simulink model "KalmanFilter_Corrected"  (R2024a)
settings: Solver=VariableStepDiscrete  StartTime=0.0  StopTime=100.0  RelTol=1e-3
values from neighbouring files (symbols this model uses):
  A = [1.1269, -0.4940, 0.1129 ... (first row only)    [KalmanFilter_Corrected_soc.m]
  B = [-0.3832,0,0 ... (first row only)    [KalmanFilter_Corrected_soc.m]
  C = [1;0;0]    [KalmanFilter_Corrected_soc.m]
  D = [0;0;0]    [KalmanFilter_Corrected_soc.m]
  P0 = eye(3)    [KalmanFilter_Corrected_soc.m]
  Q = 0    [KalmanFilter_Corrected_soc.m]
  R = [1,0, 0.1;0,0,0;0,0,0]    [KalmanFilter_Corrected_soc.m]
  X0 = [1; 0; 0]    [KalmanFilter_Corrected_soc.m]
undefined symbols (not defined in the file or in its folder): Discrete, Time
libraries: matrix_library x3, ctrlSharedLib x1
settings Model: Creator=Z634594  LastModifiedBy=DELL
settings SolverCC: AlgebraicLoopSolver=TrustRegion
settings DebuggingCC: UnconnectedInputMsg=warning  UnconnectedOutputMsg=warning  UnconnectedLineMsg=warning
settings ModelReferenceCC: EnableRefExpFcnMdlSchedulingChecks=on
settings SFSimCC: CustomCodeUndefinedFunction=UseInterfaceOnly
settings RTWCC: GPUComputeCapability=3.5

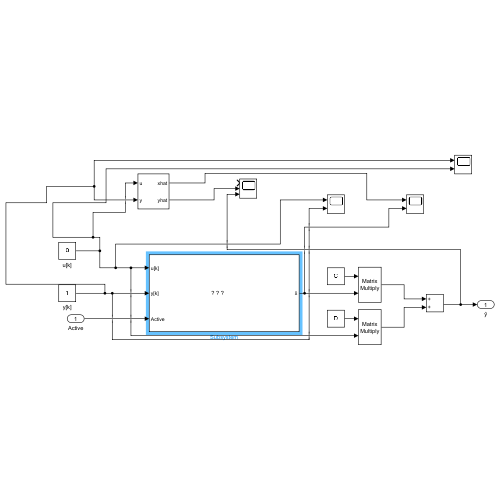
[thumbnail: Simulink's stored preview of the top-level diagram]
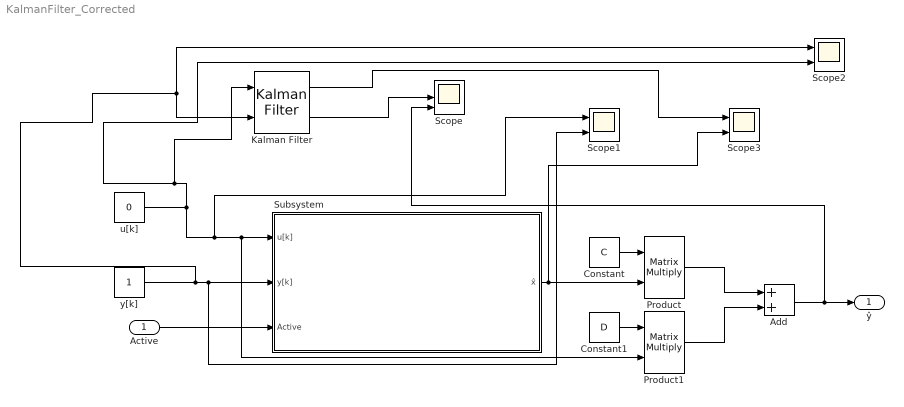
== system KalmanFilter_Corrected ==
  Active : Inport
  Add : Sum
  Constant : Constant  Value=C  VectorParams1D=off
  Constant1 : Constant  Value=D  VectorParams1D=off
  Kalman Filter : ctrlSharedLib/Kalman Filter  TimeDomain=Discrete-Time  UseCurrentEstimator=off  ModelSource=Individual A, B, C, D matrices  ModelSourceVariable=ss(0.95,1,1,0,1)  A=A  B=B  C=C  D=D  NumberOfStates=1  NumberOfInputs=1  NumberOfOutputs=1  InitialEstimateSource=Dialog  X0=[1; 0; 0];  P0=10  UseK=off  UseGH=off  NumberOfProcessNoiseInputs=1  G=1  TimeInvariantG=on  H=0  TimeInvariantH=on  Q=Q  TimeInvariantQ=on  R=1  TimeInvariantR=on  N=0  TimeInvariantN=on  AddInputPort=on  AddEnablePort=off  OutputEstimatedY=on  OutputP=off  Ts=-1
  Product : Product  Multiplication=Matrix(*)
  Product1 : Product  Multiplication=Matrix(*)
  Scope : Scope  NumInputPorts=3
  Scope1 : Scope  NumInputPorts=2
  Scope2 : Scope  NumInputPorts=2
  Scope3 : Scope  NumInputPorts=2
  Subsystem : Subsystem
      mask Display: image('C:\Users\Z634594\OneDrive - ZF Friedrichshafen AG\Workspace_MATLAB\14_Tj-Measurement\KalmanFilter\KalmanFilter\img\KalmanEquations.jpg');
  u[k] : Constant  Value=0  VectorParams1D=off
  y[k] : Constant
  ŷ : Outport  VectorParamsAs1DForOutWhenUnconnected=off
  wires:
  Active/1 -> Subsystem/3(Active)
  Subsystem/1(x̂) -> Product/2, Scope3/2
  Product1/1 -> Add/2
  Product/1 -> Add/1
  Add/1 -> Scope/3, ŷ/1
  Constant1/1 -> Product1/1
  Constant/1 -> Product/1
  u[k]/1 -> Kalman Filter/1, Scope2/2, Scope1/1, Product1/2, Subsystem/1(u[k])
  y[k]/1 -> Scope2/1, Kalman Filter/2, Scope1/2, Subsystem/2(y[k])
  Kalman Filter/2 -> Scope/2
  Kalman Filter/1 -> Scope3/1

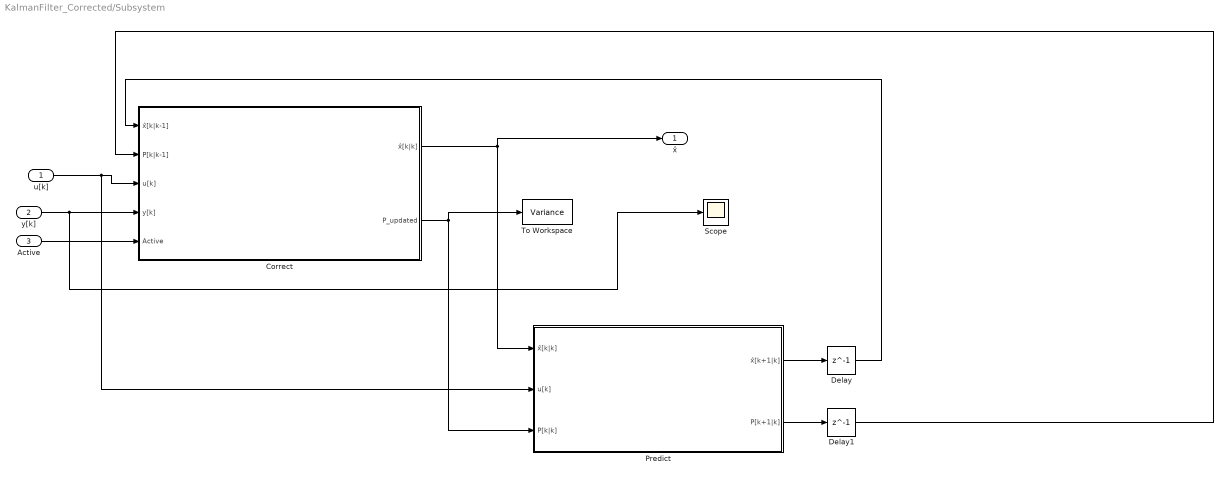
== system KalmanFilter_Corrected/Subsystem ==
  u[k] : Inport
  y[k] : Inport  Port=2
  Active : Inport  Port=3
  Correct : Subsystem
      mask Display: image('C:\Users\Z634594\OneDrive - ZF Friedrichshafen AG\Workspace_MATLAB\14_Tj-Measurement\KalmanFilter\KalmanFilter\img\Update.png');
  Delay : Delay  DelayLength=1  InitialCondition=X0
  Delay1 : Delay  DelayLength=1  InitialCondition=P0
  Predict : Subsystem
      mask Display: image('C:\Users\Z634594\OneDrive - ZF Friedrichshafen AG\Workspace_MATLAB\14_Tj-Measurement\Simulink\img\Predict.png');
  Scope : Scope
  To Workspace : ToWorkspace  VariableName=Variance  SampleTime=-1
      settings: MaxDataPoints=1
  x̂ : Outport  VectorParamsAs1DForOutWhenUnconnected=off
  wires:
  Predict/1(x̂[k+1|k]) -> Delay/1
  Delay/1 -> Correct/1(x̂[k|k-1])
  Predict/2(P[k+1|k]) -> Delay1/1
  Delay1/1 -> Correct/2(P[k|k-1])
  Correct/1(x̂[k|k]) -> x̂/1, Predict/1(x̂[k|k])
  Correct/2(P_updated) -> To Workspace/1, Predict/3(P[k|k])
  u[k]/1 -> Correct/3(u[k]), Predict/2(u[k])
  y[k]/1 -> Scope/1, Correct/4(y[k])
  Active/1 -> Correct/5(Active)

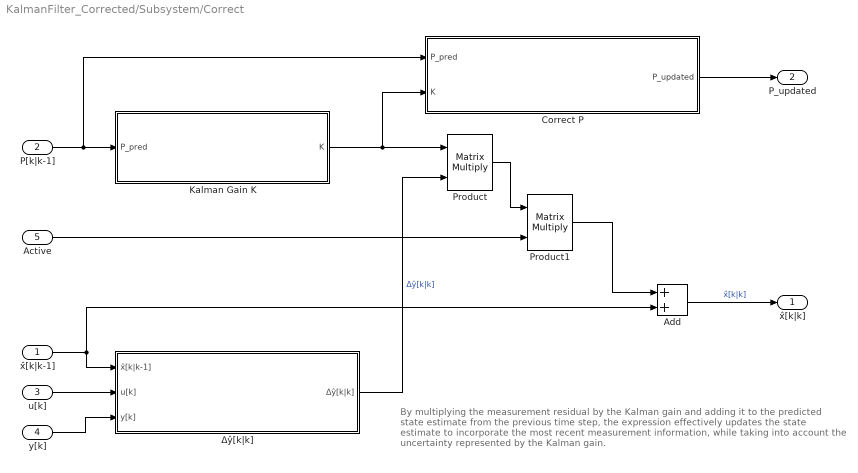
== system KalmanFilter_Corrected/Subsystem/Correct ==
  note: By multiplying the measurement residual by the Kalman gain and adding it to the predicted state estimate from the previous time step, the expression effectively updates the state estimate to incorporate the most recent measurement information, while taking into account the uncertainty represented by the Kalman gain.
  x̂[k|k-1] : Inport
  P[k|k-1] : Inport  Port=2
  u[k] : Inport  Port=3
  y[k] : Inport  Port=4
  Active : Inport  Port=5
  Add : Sum
  Correct P : Subsystem
      mask Display: image('C:\Users\Z634594\OneDrive - ZF Friedrichshafen AG\Workspace_MATLAB\14_Tj-Measurement\KalmanFilter\KalmanFilter\img\UpdateP.png');
  Kalman Gain K : Subsystem
      mask Display: image('C:\Users\Z634594\OneDrive - ZF Friedrichshafen AG\Workspace_MATLAB\14_Tj-Measurement\KalmanFilter\KalmanFilter\img\UpdateK.png');
  Product : Product  Multiplication=Matrix(*)
  Product1 : Product  Multiplication=Matrix(*)
  Δŷ[k|k] : Subsystem
      mask Display: image('C:\Users\Z634594\OneDrive - ZF Friedrichshafen AG\Workspace_MATLAB\14_Tj-Measurement\KalmanFilter\KalmanFilter\img\CalcdeltaY.png');
  x̂[k|k] : Outport  VectorParamsAs1DForOutWhenUnconnected=off
  P_updated : Outport  Port=2  VectorParamsAs1DForOutWhenUnconnected=off
  wires:
  x̂[k|k-1]/1 -> Δŷ[k|k]/1(x̂[k|k-1]), Add/2
  Add/1 -> x̂[k|k]/1  "x̂[k|k]"
  Δŷ[k|k]/1(Δŷ[k|k]) -> Product/2  "Δŷ[k|k]"
  Kalman Gain K/1(K) -> Correct P/2(K), Product/1
  P[k|k-1]/1 -> Correct P/1(P_pred), Kalman Gain K/1(P_pred)
  Correct P/1(P_updated) -> P_updated/1
  u[k]/1 -> Δŷ[k|k]/2(u[k])
  y[k]/1 -> Δŷ[k|k]/3(y[k])
  Product/1 -> Product1/1
  Product1/1 -> Add/1
  Active/1 -> Product1/2

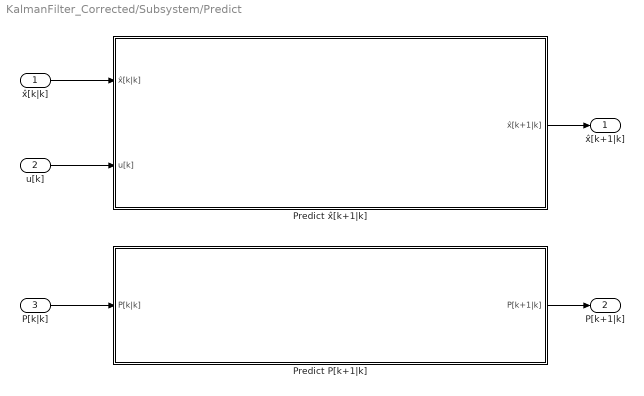
== system KalmanFilter_Corrected/Subsystem/Predict ==
  x̂[k|k] : Inport
  u[k] : Inport  Port=2
  P[k|k] : Inport  Port=3
  Predict P[k+1|k] : Subsystem
      mask Display: image('C:\Users\Z634594\OneDrive - ZF Friedrichshafen AG\Workspace_MATLAB\14_Tj-Measurement\KalmanFilter\KalmanFilter\img\PredictP.png');
  Predict x̂[k+1|k] : Subsystem
      mask Display: image('C:\Users\Z634594\OneDrive - ZF Friedrichshafen AG\Workspace_MATLAB\14_Tj-Measurement\KalmanFilter\KalmanFilter\img\Predictx.png');
  x̂[k+1|k] : Outport  VectorParamsAs1DForOutWhenUnconnected=off
  P[k+1|k] : Outport  Port=2  VectorParamsAs1DForOutWhenUnconnected=off
  wires:
  u[k]/1 -> Predict x̂[k+1|k]/2(u[k])
  x̂[k|k]/1 -> Predict x̂[k+1|k]/1(x̂[k|k])
  Predict x̂[k+1|k]/1(x̂[k+1|k]) -> x̂[k+1|k]/1
  Predict P[k+1|k]/1(P[k+1|k]) -> P[k+1|k]/1
  P[k|k]/1 -> Predict P[k+1|k]/1(P[k|k])

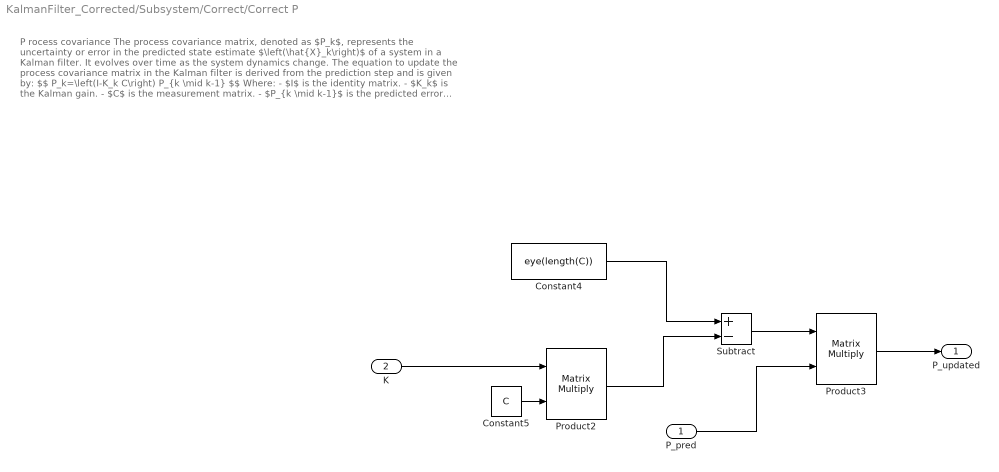
== system KalmanFilter_Corrected/Subsystem/Correct/Correct P ==
  note: P rocess covariance
      | The process covariance matrix, denoted as $P_k$, represents the uncertainty or error in the predicted state estimate $\left(\hat{X}_k\right)$ of a system in a Kalman filter. It evolves over time as the system dynamics change. The equation to update the process covariance matrix in the Kalman filter is derived from the prediction step and is given by:
      | $$
      | P_k=\left(I-K_k C\right) P_{k \mid k-1}
      | $$
      | Where:
      | - $I$ is the identity matrix.
      | - $K_k$ is the Kalman gain.
      | - $C$ is the measurement matrix.
      | - $P_{k \mid k-1}$ is the predicted error covariance matrix.
  P_pred : Inport
  K : Inport  Port=2
  Constant4 : Constant  Value=eye(length(C))  VectorParams1D=off
  Constant5 : Constant  Value=C  VectorParams1D=off
  Product2 : Product  Multiplication=Matrix(*)
  Product3 : Product  Multiplication=Matrix(*)
  Subtract : Sum  Inputs=+-
  P_updated : Outport  VectorParamsAs1DForOutWhenUnconnected=off
  wires:
  Constant5/1 -> Product2/2
  Constant4/1 -> Subtract/1
  Product2/1 -> Subtract/2
  P_pred/1 -> Product3/2
  K/1 -> Product2/1
  Subtract/1 -> Product3/1
  Product3/1 -> P_updated/1

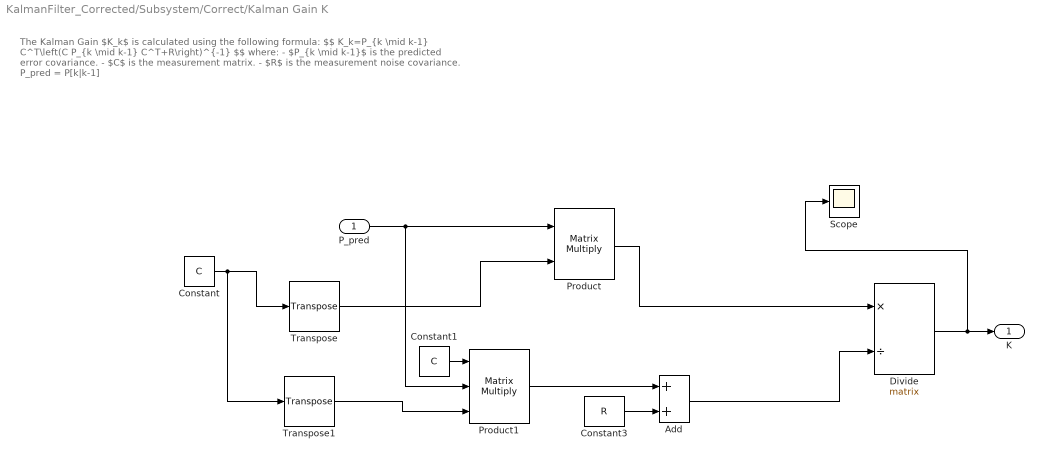
== system KalmanFilter_Corrected/Subsystem/Correct/Kalman Gain K ==
  note: The Kalman Gain $K_k$ is calculated using the following formula:
      | $$
      | K_k=P_{k \mid k-1} C^T\left(C P_{k \mid k-1} C^T+R\right)^{-1}
      | $$
      | where:
      | - $P_{k \mid k-1}$ is the predicted error covariance.
      | - $C$ is the measurement matrix.
      | - $R$ is the measurement noise covariance.
      |
      | P_pred = P[k|k-1]
  P_pred : Inport
  Add : Sum
  Constant : Constant  Value=C  VectorParams1D=off
  Constant1 : Constant  Value=C  VectorParams1D=off
  Constant3 : Constant  Value=R  VectorParams1D=off
  Divide : Product  Inputs=*/  Multiplication=Matrix(*)
  Product : Product  Multiplication=Matrix(*)
  Product1 : Product  Inputs=3  Multiplication=Matrix(*)
  Scope : Scope
  Transpose : matrix_library/Transpose
  Transpose1 : matrix_library/Transpose
  K : Outport  VectorParamsAs1DForOutWhenUnconnected=off
  wires:
  Product/1 -> Divide/1
  Constant1/1 -> Product1/1
  Divide/1 -> Scope/1, K/1
  Constant3/1 -> Add/2
  Add/1 -> Divide/2
  Product1/1 -> Add/1
  P_pred/1 -> Product1/2, Product/1
  Transpose1/1 -> Product1/3
  Transpose/1 -> Product/2
  Constant/1 -> Transpose1/1, Transpose/1

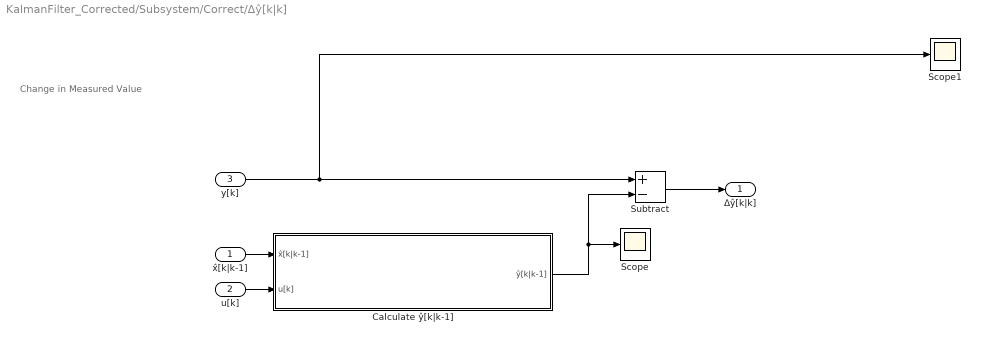
== system KalmanFilter_Corrected/Subsystem/Correct/Δŷ[k|k] ==
  note: Change in Measured Value
  x̂[k|k-1] : Inport
  u[k] : Inport  Port=2
  y[k] : Inport  Port=3
  Calculate ŷ[k|k-1] : Subsystem
      mask Display: image('C:\Users\Z634594\OneDrive - ZF Friedrichshafen AG\Workspace_MATLAB\14_Tj-Measurement\Simulink\img\Calcy.png');
  Scope : Scope
  Scope1 : Scope
  Subtract : Sum  Inputs=+-
  Δŷ[k|k] : Outport  VectorParamsAs1DForOutWhenUnconnected=off
  wires:
  x̂[k|k-1]/1 -> Calculate ŷ[k|k-1]/1(x̂[k|k-1])
  u[k]/1 -> Calculate ŷ[k|k-1]/2(u[k])
  y[k]/1 -> Scope1/1, Subtract/1
  Calculate ŷ[k|k-1]/1(ŷ[k|k-1]) -> Scope/1, Subtract/2
  Subtract/1 -> Δŷ[k|k]/1

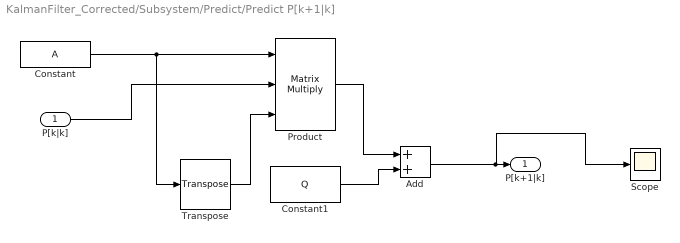
== system KalmanFilter_Corrected/Subsystem/Predict/Predict P[k+1|k] ==
  P[k|k] : Inport
  Add : Sum
  Constant : Constant  Value=A  VectorParams1D=off
  Constant1 : Constant  Value=Q  VectorParams1D=off
  Product : Product  Inputs=3  Multiplication=Matrix(*)
  Scope : Scope
  Transpose : matrix_library/Transpose
  P[k+1|k] : Outport  VectorParamsAs1DForOutWhenUnconnected=off
  wires:
  Constant/1 -> Product/1, Transpose/1
  P[k|k]/1 -> Product/2
  Product/1 -> Add/1
  Constant1/1 -> Add/2
  Add/1 -> Scope/1, P[k+1|k]/1
  Transpose/1 -> Product/3

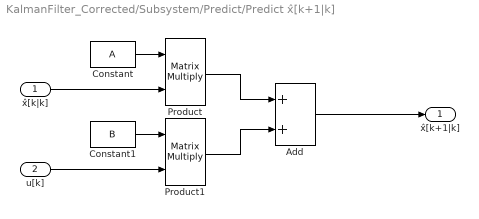
== system KalmanFilter_Corrected/Subsystem/Predict/Predict x̂[k+1|k] ==
  x̂[k|k] : Inport
  u[k] : Inport  Port=2
  Add : Sum
  Constant : Constant  Value=A  VectorParams1D=off
  Constant1 : Constant  Value=B  VectorParams1D=off
  Product : Product  Multiplication=Matrix(*)
  Product1 : Product  Multiplication=Matrix(*)
  x̂[k+1|k] : Outport  VectorParamsAs1DForOutWhenUnconnected=off
  wires:
  x̂[k|k]/1 -> Product/2
  Add/1 -> x̂[k+1|k]/1
  Constant/1 -> Product/1
  Product/1 -> Add/1
  u[k]/1 -> Product1/2
  Constant1/1 -> Product1/1
  Product1/1 -> Add/2

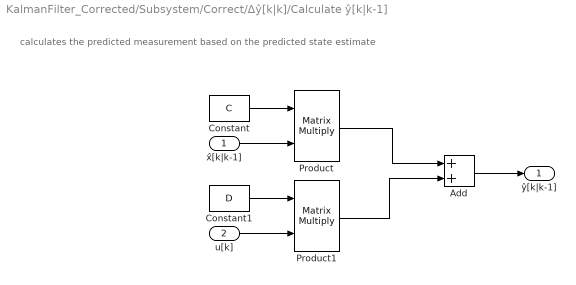
== system KalmanFilter_Corrected/Subsystem/Correct/Δŷ[k|k]/Calculate ŷ[k|k-1] ==
  note: calculates the predicted measurement based on the predicted state estimate
  x̂[k|k-1] : Inport
  u[k] : Inport  Port=2
  Add : Sum
  Constant : Constant  Value=C  VectorParams1D=off
  Constant1 : Constant  Value=D  VectorParams1D=off
  Product : Product  Multiplication=Matrix(*)
  Product1 : Product  Multiplication=Matrix(*)
  ŷ[k|k-1] : Outport  VectorParamsAs1DForOutWhenUnconnected=off
  wires:
  u[k]/1 -> Product1/2
  Product/1 -> Add/1
  x̂[k|k-1]/1 -> Product/2
  Constant/1 -> Product/1
  Constant1/1 -> Product1/1
  Add/1 -> ŷ[k|k-1]/1
  Product1/1 -> Add/2
